simulink model "Inverter"  (R2022b)
settings: Solver=VariableStepAuto  StartTime=0.0  StopTime=0.1  RelTol=1e-3
model workspace (MAT data in the model file):
  Deadtime = 1e-07
  Fsw = 6000
  Output_Freq = 60
libraries: spsMosfetLib x6, spsAsynchronousMachinepuUnitsLib x1, spsPWMGeneratorMultilevelLib x1, spsDCVoltageSourceLib x1, spsGroundLib x1, spsThreePhaseVIMeasurementLib x1, sps_lib x1
settings Model: Creator=maxim  LastModifiedBy=maxim

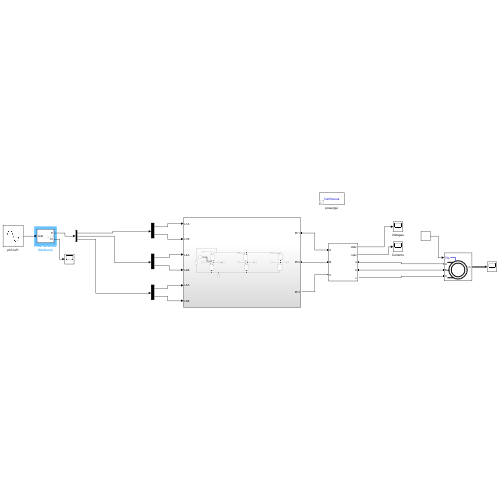
[thumbnail: Simulink's stored preview of the top-level diagram]
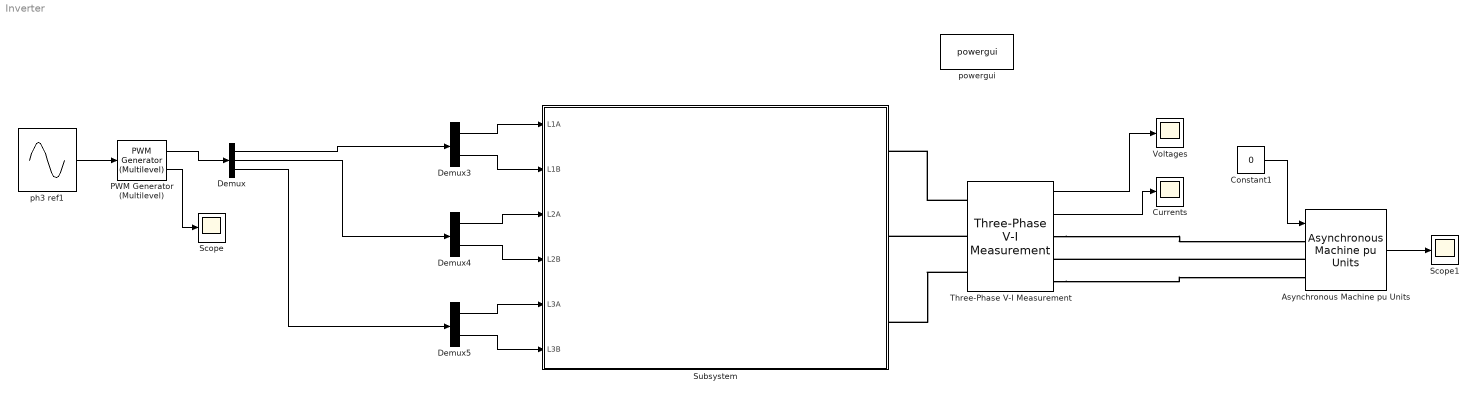
== system Inverter ==
  Asynchronous Machine pu Units : spsAsynchronousMachinepuUnitsLib/Asynchronous Machine pu Units  RotorType=Squirrel-cage  PresetModel=No  MechanicalLoad=Torque Tm  ShowDetailedParameters=on  ReferenceFrame=Rotor  Units=pu  MeasurementBus=on  NominalParameters=[3730 460 60]  VoltageRatio=1  Stator=[0.01965 0.0397]  Rotor=[0.01909 0.0397]  Cage1=[0.01909 0.0397]  Cage2=[0.01909 0.0397]  Lm=1.354  Mechanical=[0.09526 0.05479 2]  PolePairs=2  InitialConditions="[ 1,0   0,0,0   0,0,0 ]"  SimulateSaturation=off  Saturation="[0.212,0.4201,0.8125,1.0979,1.4799,2.2457,3.2586,4.5763,6.4763 ;   0.5,0.7,0.9,1,1.1,1.2 ,1.3,1.4,1.5]"  LoadFlowParameters=0  TsPowergui=0  TsBlock=-1  IterativeModel=Trapezoidal non iterative  IterativeDiscreteModel=Trapezoidal non iterative  Pmec=0
      settings: LibrarySourceBlock=|
      | sps_lib/Electrical Machines/Asynchronous Machine
      | pu Units
  Constant1 : Constant  Value=0
  Currents : Scope
  Demux : Demux  Outputs=3
  Demux3 : Demux  Outputs=2
  Demux4 : Demux  Outputs=2
  Demux5 : Demux  Outputs=2
  PWM Generator (Multilevel) : spsPWMGeneratorMultilevelLib/PWM Generator (Multilevel)  BridgeType=Half-bridge  NumberOfBridges=3  Fc=Fsw  Ts=0  ShowCarriersOutport=on
      settings: LibrarySourceBlock=|
      | sps_lib/Power Electronics/Power Electronics Control/PWM Generator
      | (Multilevel)
  Scope : Scope
  Scope1 : Scope
  Subsystem : Subsystem
  Three-Phase V-I Measurement : spsThreePhaseVIMeasurementLib/Three-Phase V-I Measurement  VoltageMeasurement=phase-to-ground  SetLabelV=off  LabelV=Vabc  Vpu=off  VpuLL=off  CurrentMeasurement=yes  SetLabelI=off  LabelI=Iabc  Ipu=off  Pbase=100e6  Vbase=500e3  OutputType=Complex  PhasorSimulation=off  PSBequivalent=0
  Voltages : Scope
  ph3 ref1 : Sin  Amplitude=1/2  Bias=1/2  Frequency=Output_Freq  SampleTime=0
  powergui : sps_lib/powergui  Priority=1  SimulationMode=Continuous  SampleTime=50e-6  frequency=60  Iterations=50  frequencyindice=0  Pbase=100e6  ErrMax=1e-4  UnitsV=kV  UnitsW=MW  buscounter=0  FunctionMessages=off  echomessages=off  EnableUseOfTLC=off  CurrentSourceSwitches=off  DisableSnubberDevices=off  DisableRonSwitches=off  DisableVfSwitches=off  DisplayEquations=off  AutomaticDiscreteSolvers=off  SolverType=Tustin/Backward Euler (TBE)  Interpol=off  ExternalGateDelay=off  methode=off  Ts=100  x0status=blocks  SPID=on  SwTol=0  HookPort=off  NonlinearTolerance=1e-4  nMaxIteration=100  ContinueOnMaxIteration=off  RestoreLinks=warning  ResistiveCurrentMeasurement=off  Frange=[0:2:500]  Ylog=off  Xlog=on  ShowGrid=off  save=off  variable=ZData  structure=0  ZoomFFT=off  StartTime=0.0  cycles=1  DisplayStyle=1  fundamental=60  FreqAxis=off  MaxFrequency=1000  frequencyindicesteady=1  RmsSteady=1  display=off
  wires:
  Demux3/1 -> Subsystem/1(L1A)
  Demux3/2 -> Subsystem/2(L1B)
  Demux4/1 -> Subsystem/3(L2A)
  Demux4/2 -> Subsystem/4(L2B)
  Demux5/1 -> Subsystem/5(L3A)
  Demux5/2 -> Subsystem/6(L3B)
  Constant1/1 -> Asynchronous Machine pu Units/1
  Asynchronous Machine pu Units/1 -> Scope1/1
  Three-Phase V-I Measurement/1 -> Voltages/1
  Three-Phase V-I Measurement/2 -> Currents/1
  ph3 ref1/1 -> PWM Generator (Multilevel)/1
  PWM Generator (Multilevel)/1 -> Demux/1
  Demux/1 -> Demux3/1
  Demux/2 -> Demux4/1
  Demux/3 -> Demux5/1
  PWM Generator (Multilevel)/2 -> Scope/1
  connections:
  Three-Phase V-I Measurement/LConn2 -- Subsystem/RConn2
  Three-Phase V-I Measurement/LConn1 -- Subsystem/RConn1
  Three-Phase V-I Measurement/LConn3 -- Subsystem/RConn3
  Three-Phase V-I Measurement/RConn1 -- Asynchronous Machine pu Units/LConn1
  Asynchronous Machine pu Units/LConn2 -- Three-Phase V-I Measurement/RConn2
  Three-Phase V-I Measurement/RConn3 -- Asynchronous Machine pu Units/LConn3

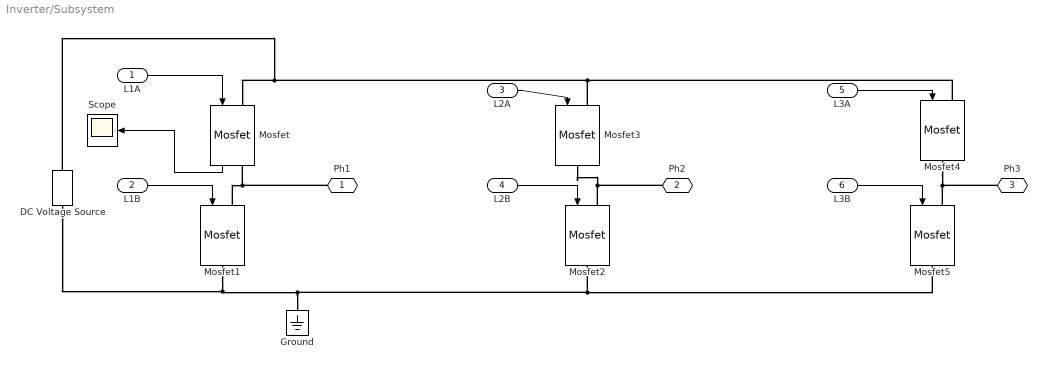
== system Inverter/Subsystem ==
  L1A : Inport
  L1B : Inport  Port=2
  L2A : Inport  Port=3
  L2B : Inport  Port=4
  L3A : Inport  Port=5
  L3B : Inport  Port=6
  DC Voltage Source : spsDCVoltageSourceLib/DC Voltage Source  Amplitude=100  Measurements=None
  Ground : spsGroundLib/Ground  LConnTagsString=a
  Mosfet : spsMosfetLib/Mosfet  Ron=0.01  Lon=0  Rd=0.01  Vfd=0.7  IC=0  Rs=0.2  Cs=1e-9  Measurements=on
  Mosfet{1..3,5} (4 alike) : spsMosfetLib/Mosfet  Ron=0.01  Lon=0  Rd=0.01  Vfd=0.7  IC=0  Rs=0.2  Cs=1e-9  Measurements=off
  Mosfet4 : spsMosfetLib/Mosfet  Ron=0.01  Lon=0  Rd=0.01  Vfd=0.7  IC=0  Rs=0.  Cs=1e-9  Measurements=off
  Scope : Scope
  Ph1 : PMIOPort  Side=Right
  Ph2 : PMIOPort  Port=2  Side=Right
  Ph3 : PMIOPort  Port=3  Side=Right
  wires:
  L1A/1 -> Mosfet/1
  L2A/1 -> Mosfet3/1
  L2B/1 -> Mosfet2/1
  L3B/1 -> Mosfet5/1
  L3A/1 -> Mosfet4/1
  L1B/1 -> Mosfet1/1
  Mosfet/1 -> Scope/1
  connections:
  Mosfet/RConn1 -- Mosfet1/LConn1 -- Ph1/RConn1
  Ground/LConn1 -- DC Voltage Source/LConn1 -- Mosfet1/RConn1 -- Mosfet5/RConn1 -- Mosfet2/RConn1
  Ph2/RConn1 -- Mosfet3/RConn1 -- Mosfet2/LConn1
  Mosfet4/LConn1 -- Mosfet3/LConn1 -- DC Voltage Source/RConn1 -- Mosfet/LConn1
  Ph3/RConn1 -- Mosfet5/LConn1 -- Mosfet4/RConn1
